simulink model "dsplpc"  (Simulink 6.0)
settings: Solver=FixedStepDiscrete  SolverMode=SingleTasking  StartTime=0.0  StopTime=0.49  RelTol=1e-3
PreLoadFcn:
  | load mtlb;
undefined symbols (not defined in the file or in its folder): Mag, mtlb
libraries: dsparch4 x4, dspsnks4 x3, dspsigops x2, dspsrcs4 x1, dspstat3 x1, dspxfrm3 x1, dspsolvers x1, dspbuff3 x1
settings Model: RequirementInfo=9  CovMetricSettings=d  Creator=dshpak  LastModifiedBy=mlongfri  ExtModeTrigMode=oneshot  ExtModeArmWhenConnect=off  ExtModeAutoUpdateStatusClock=off  ProdHWDeviceType=Specified
settings DataIOCC: LimitDataPoints=off  SaveFormat=Structure  SaveOutput=off  SaveTime=off  SignalLoggingName=sigsOut
settings OptimizationCC: BlockReduction=off  BooleanDataType=off  InlineInvariantSignals=off  MultiInstanced=off
settings FormatCC: IgnoreBidirectionalLines=off
settings DebuggingCC: IntegerOverflowMsg=none
settings HardwareCC: ProdHWDeviceType=Specified
settings CodeAppCC: SimulinkBlockComments=off
settings GRTTargetCC: TargetFcnLib=iso_c_tmw.mat

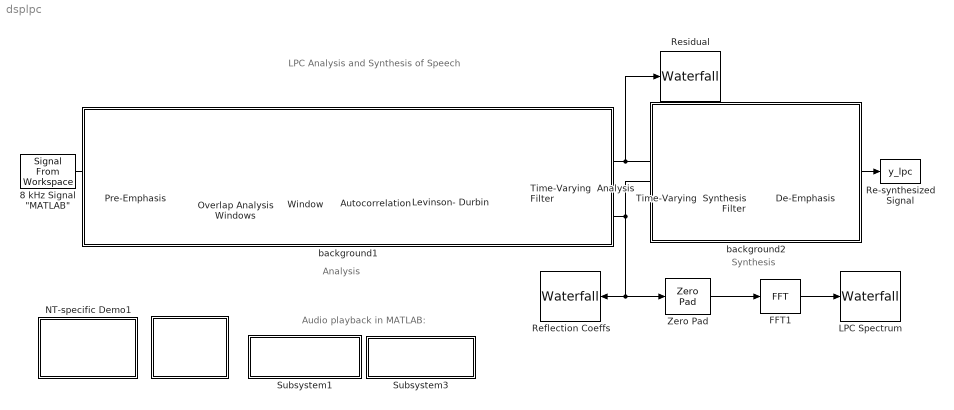
== system dsplpc ==
  note: LPC Analysis and Synthesis of Speech
  note: Analysis
  note: Synthesis
  note: Audio playback in MATLAB:
  " " : Subsystem
      mask Type: Frame-Based Simulation Info
      mask Display: disp('Info')
  "8 kHz Signal \"MATLAB\"" : dspsrcs4/Signal From Workspace  X=mtlb*0.32  Ts=1/8000  nsamps=80  OutputAfterFinalValue=Setting to zero
  Autocorrelation : dspstat3/Autocorrelation  DialogController=dspDDGCreate  DialogControllerArgs=DataTag0  AllPositiveLags=off  maxlag=12  bias=Biased  domain=Time  roundingMode=Floor  overflowMode=off
  De-Emphasis : dsparch4/Digital Filter  TypePopup=IIR (all poles)  IIRFiltStruct=Direct form II transposed  AllPoleFiltStruct=Direct form  FIRFiltStruct=Direct form  CoeffSource=Specify via dialog  NumCoeffs=[1 -.95]  DenCoeffs=[1 -.95]  BiQuadCoeffs=[1 0.3 0.4 1 0.1 0.2]  LatticeCoeffs=[0.2 0.4]  denIgnore=on  FiltPerSampPopup=One filter per frame  IC=0  ICnum=0  ICden=0  roundingMode=Floor  overflowMode=off
  FFT1 : dspxfrm3/FFT  DialogController=dspDDGCreate  DialogControllerArgs=DataTag1  CompMethod=Table lookup  TableOpt=Speed  BitRevOrder=off  SkipNorm=off  roundingMode=Floor  overflowMode=off
  LPC Spectrum : dspsnks4/Waterfall  TraceProperties=off  NumTraces=10  CMapStr=autumn  TNewest=0.35  TOldest=0.1  HistoryLength=100  HistoryFull=Overwrite  UpdateInterval=1  ExportMode=All visible  MLExportName=ExportData  AutoExport=off  DisplayProperties=off  MouseMode=Orbit  AxisGrid=off  Snapshot=off  Suspend=off  SyncSnapshots=off  OpenScopeAtSimStart=on  FigPos=[452 44 407 353]  CameraView=[89945.9047576273 49093.2447020758 -7462.52930692949 -16.6995606364064 71 5.5 2.5389885178677 -5.30668596526891 0.808418434368868 0.0592442608385446 5.583225828012 14.2 1]  InportDimsHint=[129 1]  AxisProperties=off  AxisColor=[1 1 1]*.9  XLabel=Frequency  YLabel=Mag^2  ZLabel=History  TriggerProperties=off  TrigStartMode=Immediately  TrigStartT=10  TrigStartN=1000  TrigStartFcn=trigPower  TrigStopMode=Never  TrigStopT=0.1  TrigStopN=10  TrigStopFcn=trigend  TrigRearmMode=User-defined  TrigRearmT=0  TrigRearmN=100  TrigRearmFcn=trigrearm  XformProperties=off  XformMode=FFT->Mag dB Fs/2  XformFcn=fliplr  XformExpr=20*log10(abs(u(129:2:end)))
      settings: YMin=-44.6156897764664  YMax=11.2165685036536
  Levinson- Durbin : dspsolvers/Levinson-Durbin  DialogController=dspDDGCreate  DialogControllerArgs=DataTag2  coeffOutFcn=K  outP=off  zeroInpHandling=on  firstCoeffMode=Binary point scaling  firstCoeffWordLength=16  firstCoeffFracLength=15  secondCoeffMode=Binary point scaling  secondCoeffWordLength=16  secondCoeffFracLength=15  roundingMode=Floor  overflowMode=off
      settings: allowOverrides=off
  NT-specific Demo1 : Subsystem
      settings: OpenFcn=dsplpc_win32
      mask Type: NT-only Demo
      mask Display: disp('PC/Windows\nLPC Demo')
  Overlap Analysis Windows : dspbuff3/Buffer  N=160  V=80  ic=0
  Pre-Emphasis : dsparch4/Digital Filter  TypePopup=FIR (all zeros)  IIRFiltStruct=Direct form II transposed  AllPoleFiltStruct=Direct form  FIRFiltStruct=Direct form  CoeffSource=Specify via dialog  NumCoeffs=[1 -.95]  DenCoeffs=[1 0.1]  BiQuadCoeffs=[1 0.3 0.4 1 0.1 0.2]  LatticeCoeffs=[0.2 0.4]  denIgnore=on  FiltPerSampPopup=One filter per frame  IC=0  ICnum=0  ICden=0  roundingMode=Floor  overflowMode=off
  Re-synthesized Signal : ToWorkspace  VariableName=y_lpc  SampleTime=-1  SaveFormat=Array
  Reflection Coeffs : dspsnks4/Waterfall  Orientation=left  TraceProperties=off  NumTraces=10  CMapStr=autumn  TNewest=0.7  TOldest=0.1  HistoryLength=50  HistoryFull=Overwrite  UpdateInterval=1  ExportMode=All visible  MLExportName=ExportData2  AutoExport=off  DisplayProperties=off  MouseMode=Orbit  AxisGrid=on  Snapshot=off  Suspend=off  SyncSnapshots=off  OpenScopeAtSimStart=on  FigPos=[35 41 410 358]  CameraView=[73343.0440471642 150383.489958622 -231607.055769344 -0.0735265549347769 7.5 5.5 0.547487828138618 -2.62241953831449 4.03911084299836 0.00240035045613671 1 7.88928028685195 5.25952019123463]  InportDimsHint=[12 1]  AxisProperties=off  AxisColor=[1 1 1]*.9  XLabel=Coefficient  YLabel=RC Amplitude  ZLabel=History  TriggerProperties=off  TrigStartMode=Immediately  TrigStartT=10  TrigStartN=1000  TrigStartFcn=trigPower  TrigStopMode=Never  TrigStopT=0.1  TrigStopN=10  TrigStopFcn=trigend  TrigRearmMode=User-defined  TrigRearmT=0  TrigRearmN=100  TrigRearmFcn=trigrearm  XformProperties=off  XformMode=None  XformFcn=fliplr  XformExpr=20*log10(abs(u(129:2:end)))
      settings: YMin=-1.02418361455266  YMax=0.877130504683106
  Residual : dspsnks4/Waterfall  TraceProperties=off  NumTraces=10  CMapStr=autumn  TNewest=0.7  TOldest=0.1  HistoryLength=50  HistoryFull=Overwrite  UpdateInterval=1  ExportMode=All visible  MLExportName=ExportData2  AutoExport=off  DisplayProperties=off  MouseMode=Orbit  AxisGrid=on  Snapshot=off  Suspend=off  SyncSnapshots=off  OpenScopeAtSimStart=off  FigPos=[524 276 410 358]  CameraView=[62164.2347969079 1792549.89917746 -405278.370332737 -0.097024155318337 44.5 5.5 0.575539043328793 -33.5051317778483 7.57548038023531 0.00104183380472551 1 92.0645761641202 10.3443344004629]  InportDimsHint=[80 1]  AxisProperties=off  AxisColor=[1 1 1]*.9  XLabel=Coefficient  YLabel=Amplitude  ZLabel=History  TriggerProperties=off  TrigStartMode=Immediately  TrigStartT=10  TrigStartN=1000  TrigStartFcn=trigPower  TrigStopMode=Never  TrigStopT=0.1  TrigStopN=10  TrigStopFcn=trigend  TrigRearmMode=User-defined  TrigRearmT=0  TrigRearmN=100  TrigRearmFcn=trigrearm  XformProperties=off  XformMode=None  XformFcn=fliplr  XformExpr=20*log10(abs(u(129:2:end)))
      settings: YMin=-0.580380532484202  YMax=0.386332221847528
  Subsystem1 : Subsystem
      settings: OpenFcn=if exist('mtlb','var'), sound(mtlb*0.32,8000); else errordlg('Data not found in workspace - reload demo model.','Signal Processing Blockset Demo Error'); end
      mask Display: disp('Original\nSignal')
  Subsystem3 : Subsystem
      settings: OpenFcn=if exist('y_lpc','var'), sound(y_lpc,8000); else errordlg('You must run the simulation first.','Signal Processing Blockset Demo Error'); end
      mask Display: disp('Processed\nSignal')
  Time-Varying  Analysis Filter : dsparch4/Digital Filter  TypePopup=FIR (all zeros)  IIRFiltStruct=Direct form II transposed  AllPoleFiltStruct=Direct form  FIRFiltStruct=Lattice MA  CoeffSource=Input port(s)  NumCoeffs=[1 -.95]  DenCoeffs=[1 0.1]  BiQuadCoeffs=[1 0.3 0.4 1 0.1 0.2]  LatticeCoeffs=[0.2 0.4]  denIgnore=on  FiltPerSampPopup=One filter per frame  IC=0  ICnum=0  ICden=0  roundingMode=Floor  overflowMode=off
  Time-Varying  Synthesis Filter : dsparch4/Digital Filter  TypePopup=IIR (all poles)  IIRFiltStruct=Direct form II transposed  AllPoleFiltStruct=Lattice AR  FIRFiltStruct=Direct form  CoeffSource=Input port(s)  NumCoeffs=[1 -.95]  DenCoeffs=[1 0.1]  BiQuadCoeffs=[1 0.3 0.4 1 0.1 0.2]  LatticeCoeffs=[0.2 0.4]  denIgnore=on  FiltPerSampPopup=One filter per frame  IC=0  ICnum=0  ICden=0  roundingMode=Floor  overflowMode=off
  Window : dspsigops/Window Function  winmode=Apply window to input  wintype=Hamming  sampmode=Continuous  samptime=1  N=64  Rs=50  beta=10  winsamp=Symmetric  UserWindow=hamming  OptParams=off  UserParams={1.0}  dataType=double  isSigned=on  wordLen=16  udDataType=sfix(16)  fracBitsMode=Best precision  numFracBits=15  roundingMode=Floor  overflowMode=off
  Zero Pad : dspsigops/Zero Pad  padSigAt=End  zpadAlong=Columns  padNumOutRowsSpecMethod=User-specified  numOutRows=256  padNumOutColsSpecMethod=User-specified  numOutCols=1  trunc_flag=None
  background1 : Subsystem
      mask Display: disp('')
  background2 : Subsystem
      mask Display: disp('')
  wires:
  "8 kHz Signal \"MATLAB\""/1 -> Pre-Emphasis/1
  Pre-Emphasis/1 -> Overlap Analysis Windows/1, Time-Varying  Analysis Filter/1
  Overlap Analysis Windows/1 -> Window/1
  Autocorrelation/1 -> Levinson- Durbin/1
  Window/1 -> Autocorrelation/1
  Time-Varying  Analysis Filter/1 -> Time-Varying  Synthesis Filter/1, Residual/1
  Levinson- Durbin/1 -> Time-Varying  Synthesis Filter/2, Reflection Coeffs/1, Zero Pad/1, Time-Varying  Analysis Filter/2
  Time-Varying  Synthesis Filter/1 -> De-Emphasis/1
  De-Emphasis/1 -> Re-synthesized Signal/1
  Zero Pad/1 -> FFT1/1
  FFT1/1 -> LPC Spectrum/1

== system dsplpc/  ==
  note: LPC Analysis and Synthesis of Speech
      |
      | This demo consists of two parts,  analysis and synthesis. The analysis part
      | is found in the transmitter section of a system. Using the original speech signal, parameters
      | (reflection coefficients) and the residual signal are extracted from it, and then transmitted over
      | a channel. The synthesis part , which is found in the receiver section of the system, reconstructs
      | the original signal using those parameters and the residual signal.
      |
      | In this simulation , the speech signal is divided into
      | frames of size 20 ms (160 samples) , with an overlap of 10 ms (80 samples).Each frame
      | is then windowed using a hamming window, 11th order autocorrelation coefficients
      | are found and then the reflection coefficients (11th order) are calculated from the autocorrelation
      | coefficients, using the Levinson-Durbin algorithm. The original speech signal is passed through an
      |  analysis-filter which is basically an all-zero filter with coefficients as the reflection coefficients
      | obtained above. The output of the filter is the residual signal. This residual signal is then
      | passed through a synthesis-filter which is basically an all-pole filter, again with coefficients as the
      | reflection coefficients (Synthesis filter is just the inverse of Analysis filter). The output of the
      | synthesis filter is the original signal.

== system dsplpc/NT-specific Demo1 ==

== system dsplpc/Subsystem1 ==

== system dsplpc/Subsystem3 ==

== system dsplpc/background1 ==

== system dsplpc/background2 ==
